simulink model "zynqRadioQPSKRxFPGAAD9361AD9364RetargetSL"  (R2016a)
settings: Solver=FixedStepDiscrete  SolverMode=SingleTasking  StartTime=0.0  StopTime=inf  RelTol=1e-3
PreLoadFcn:
  | sdrzQPSKRxFPGAretarget_params =zynqRadioQPSKRxFPGAAD9361AD9364SL_init;
InitFcn:
  | sdrzQPSKRxFPGAretarget_params = zynqRadioQPSKRxFPGAAD9361AD9364SL_init;
undefined symbols (not defined in the file or in its folder): F
libraries: hdlsllib x3, sdrzblksprivate x1, commsequence2 x1, zc706fmc234_lib x1
CloseFcn:
  | clear sdrzQPSKRxFPGAretarget_params;
Description:
  | This model uses a targeted .bit generated from the sdrzQPSKRxFPGAFMC234 example to receive a QPSK signal using SDR hardware
settings Model: FPTRunName=Active  ModifiedByFormat=The MathWorks Inc.  SimulationMode=accelerator  Creator=The MathWorks, Inc.  LastModifiedBy=The MathWorks Inc.
settings DataIOCC: LimitDataPoints=on  SaveFormat=Structure  SaveOutput=off  SignalLogging=off  DSMLogging=off  SaveTime=off
settings OptimizationCC: BlockReduction=off  ConditionallyExecuteInputs=off  DefaultParameterBehavior=Inlined  ExpressionDepthLimit=2147483647  LocalBlockOutputs=off  SimCompilerOptimization=on
settings DebuggingCC: AlgebraicLoopMsg=error  UnderspecifiedInitializationDetection=Classic  MergeDetectMultiDrivingBlocksExec=none  SolverPrmCheckMsg=warning  MultiTaskDSMMsg=warning  MultiTaskCondExecSysMsg=none  SingleTaskRateTransMsg=error  ParameterPrecisionLossMsg=none  FcnCallInpInsideContextMsg=UseLocalSettings  AllowSymbolicDim=off  StateNameClashWarn=warning
settings HardwareCC: ProdBitPerPointer=32  ProdLargestAtomicFloat=None  ProdIntDivRoundTo=Undefined  ProdEndianess=Unspecified  ProdWordSize=32  ProdHWDeviceType=ASIC/FPGA->ASIC/FPGA  TargetBitPerPointer=64  TargetLongLongMode=on  TargetIntDivRoundTo=Zero  TargetEndianess=LittleEndian  TargetWordSize=64  TargetHWDeviceType=MATLAB Host  ProdEqTarget=off
settings ModelReferenceCC: PropagateSignalLabelsOutOfModel=off
settings RTWCC: CustomSourceCode=|
  | #include <stdio.h>
  | #include <stdlib.h>
settings GRTTargetCC: CombineOutputUpdateFcns=off  GRTInterface=on
settings ConfigComp: CovModelRefEnable=Off  CovSFcnEnable=off

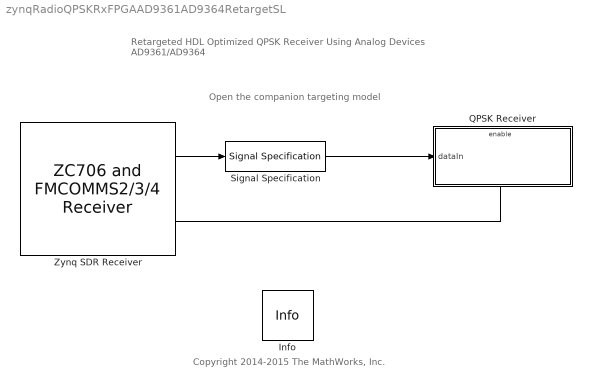
== system zynqRadioQPSKRxFPGAAD9361AD9364RetargetSL ==
  note: Copyright 2014-2015 The MathWorks, Inc.
  note: Retargeted HDL Optimized QPSK Receiver
      | Using Analog Devices AD9361/AD9364
  note: Open the companion targeting model
  Info : sdrzblksprivate/Info  SystemSampleTime=-1
  QPSK Receiver : Subsystem
      mask Display: disp('QPSK Receiver')
  Signal Specification : SignalSpecification  SampleTime=sdrzQPSKRxFPGAretarget_params.Upsampling*sdrzQPSKRxFPGAretarget_params.FrameSize*sdrzQPSKRxFPGAretarget_params.RxBufferedFrames/sdrzQPSKRxFPGAretarget_params.RadioFrontEndSampleRate
  Zynq SDR Receiver : zc706fmc234_lib/ZC706 and  FMCOMMS2//3//4  Receiver  IPAddress=192.168.3.2  CenterFrequencySource=Dialog  CenterFrequency=sdrzQPSKRxFPGAretarget_params.RadioCenterFrequency  GainSource=AGC Slow Attack  Gain=1  ChannelMapping=1  BasebandSampleRate=sdrzQPSKRxFPGAretarget_params.RadioFrontEndSampleRate  EnableBurstMode=on  NumFramesInBurst=20  OutputDataType=int16  SamplesPerFrame=sdrzQPSKRxFPGAretarget_params.Upsampling*sdrzQPSKRxFPGAretarget_params.FrameSize*sdrzQPSKRxFPGAretarget_params.RxBufferedFrames  LostSamplesOutputPort=off  RSSIOutputPort=off  DMATimeoutValue=1  blockMode=Normal  EnableQuadratureTracking=on  EnableRFDCTracking=on  EnableBasebandDCTracking=on  BypassUserLogic=off  ShowAdvancedProperties=on  ShowInternalProperties=off  subDeviceList=zynqReceiver  sdrExecutionMode=HW  dataUDPPort=-1  ctrlUDPPort=-1  SourceSelect=RF data  SourceConfiguration1=1023  FIRCoefficientSize=[ 128; 128 ]  FIRCoefficients=[ 111, -87, 147, -127, -18, -286, -312, -555, -601, -722, -642, -555, -303, -66, 221, 393, 488, 403, 219, -74, -343, -550, -582, -450, -146, 221, 569, 759, 735, 463, 20, -487, -885, -1048, -883, -418, 243, 897, 1340, 1394, 1002, 228, -715, -1549, -1980, -1819, -1028, 217, 1583, 2635, 2980, 2377, 853, -1275, -3435, -4926, -5080, -3454, 40, 5065, 10903, 16581, 21085, 23573, 23573, 21085, 16581, 10903, 5065, 40, -3454, -5080, -4926, -3435, -1275, 853, 2377, 2980, 2635, 1583, 217, -1028, -1819, -1980, -1549, -715, 228, 1002, 1394, 1340, 897, 243, -418, -883, -1048, -885, -487, 20, 463, 735, 759, 569, 221, -146, -450, -582, -550, -343, -74, 219, 403, 488, 393, 221, -66, -303, -555, -642, -722, -601, -555, -312, -286, -18, -127, 147, -87, 111; 382, -200, 711, -41, 645, 36, 346, -194, -119, -543, -472, -646, -404, -312, 45, 197, 413, 346, 241, -93, -373, -680, -755, -689, -356, 51, 515, 795, 870, 609, 136, -488, -1009, -1303, -1191, -712, 69, 885, 1516, 1692, 1336, 468, -662, -1740, -2378, -2329, -1494, -55, 1620, 2995, 3584, 3045, 1368, -1121, -3755, -5708, -6156, -4542, -710, 4969, 11669, 18243, 23486, 26391, 26391, 23486, 18243, 11669, 4969, -710, -4542, -6156, -5708, -3755, -1121, 1368, 3045, 3584, 2995, 1620, -55, -1494, -2329, -2378, -1740, -662, 468, 1336, 1692, 1516, 885, 69, -712, -1191, -1303, -1009, -488, 136, 609, 870, 795, 515, 51, -356, -689, -755, -680, -373, -93, 241, 346, 413, 197, 45, -312, -404, -646, -472, -543, -119, -194, 346, 36, 645, -41, 711, -200, 382 ]  FIRGain=[ 0; -12 ]  FIRDecimInterpFactor=[ 4; 4 ]  AnalogFilterCutoff=[ 2560000; 2560000 ]  FilterPathRates=[ 737280000, 184320000, 61440000, 30720000, 15360000, 3840000; 737280000, 184320000, 61440000, 30720000, 15360000, 3840000 ]  FilterDesignTypeForTx=DefaultFilterFromOther  FilterDesignTypeForRx=DefaultFilter  BISTLoopbackConfig=No Loopback  BISTPRBSMode=PRBS Disable  BISTToneMode=Tone Disable  BISTToneFrequency=F/32  BISTToneLevel=-6  BISTChannelMask=0  DataIsComplex=on  SimulateUsing=Code generation
  wires:
  Zynq SDR Receiver/2 -> QPSK Receiver/Enable
  Zynq SDR Receiver/1 -> Signal Specification/1
  Signal Specification/1 -> QPSK Receiver/1(dataIn)

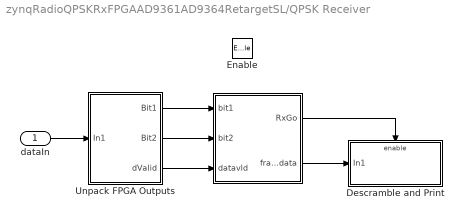
== system zynqRadioQPSKRxFPGAAD9361AD9364RetargetSL/QPSK Receiver ==
  dataIn : Inport  OutDataTypeStr=int16
  Enable : EnablePort
  " " : MATLAB Function  TreatAsAtomicUnit=on
  Descramble and Print : Subsystem  TreatAsAtomicUnit=on
  Unpack FPGA Outputs : Subsystem
  wires:
  Unpack FPGA Outputs/2(Bit2) -> " "/2(bit2)
  Unpack FPGA Outputs/1(Bit1) -> " "/1(bit1)
  Unpack FPGA Outputs/3(dValid) -> " "/3(datavld)
  dataIn/1 -> Unpack FPGA Outputs/1(In1)
  " "/1(RxGo) -> Descramble and Print/Enable
  " "/2(framed_data) -> Descramble and Print/1(In1)

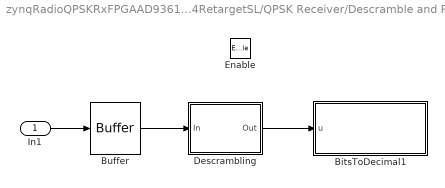
== system zynqRadioQPSKRxFPGAAD9361AD9364RetargetSL/QPSK Receiver/Descramble and Print ==
  In1 : Inport
  Enable : EnablePort
  BitsToDecimal1 : MATLAB Function  TreatAsAtomicUnit=on
  Buffer : Buffer  N=200  TreatMby1Signals=One channel  OutputFrames=off
  Descrambling : Subsystem
      mask Display: disp('Descrambling')
  wires:
  Descrambling/1(Out) -> BitsToDecimal1/1(u)
  In1/1 -> Buffer/1
  Buffer/1 -> Descrambling/1(In)

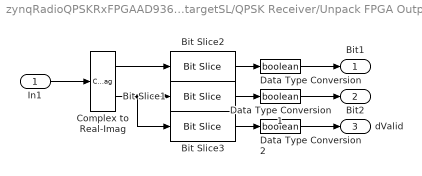
== system zynqRadioQPSKRxFPGAAD9361AD9364RetargetSL/QPSK Receiver/Unpack FPGA Outputs ==
  In1 : Inport
  Bit Slice1 : hdlsllib/HDL Operations/Bit Slice  lidx=0  ridx=0
  Bit Slice2 : hdlsllib/HDL Operations/Bit Slice  lidx=0  ridx=0
  Bit Slice3 : hdlsllib/HDL Operations/Bit Slice  lidx=15  ridx=15
  Complex to Real-Imag : ComplexToRealImag
  Data Type Conversion : DataTypeConversion  OutDataTypeStr=boolean
  Data Type Conversion1 : DataTypeConversion  OutDataTypeStr=boolean
  Data Type Conversion2 : DataTypeConversion  OutDataTypeStr=boolean
  Bit1 : Outport
  Bit2 : Outport  Port=2
  dValid : Outport  Port=3
  wires:
  In1/1 -> Complex to Real-Imag/1
  Complex to Real-Imag/1 -> Bit Slice2/1
  Complex to Real-Imag/2 -> Bit Slice3/1, Bit Slice1/1
  Bit Slice2/1 -> Data Type Conversion/1
  Bit Slice1/1 -> Data Type Conversion1/1
  Bit Slice3/1 -> Data Type Conversion2/1
  Data Type Conversion/1 -> Bit1/1
  Data Type Conversion1/1 -> Bit2/1
  Data Type Conversion2/1 -> dValid/1

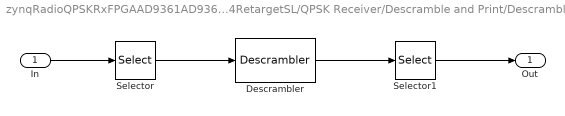
== system zynqRadioQPSKRxFPGAAD9361AD9364RetargetSL/QPSK Receiver/Descramble and Print/Descrambling ==
  In : Inport
  Descrambler : commsequence2/Descrambler  M=2  poly=[1 1 1 0 1]  iniStaSource=Dialog Parameter  ini_sta=[0 0 0 0]  resetViaPort=off
  Selector : Selector  IndexOptions=Index vector (dialog)  Indices=[sdrzQPSKRxFPGAretarget_params.BarkerLength*log2(sdrzQPSKRxFPGAretarget_params.M)+1:sdrzQPSKRxFPGAretarget_params.FrameSize*log2(sdrzQPSKRxFPGAretarget_params.M)]  OutputSizes=1
  Selector1 : Selector  IndexOptions=Index vector (dialog)  Indices=[1:sdrzQPSKRxFPGAretarget_params.MsgLength]  OutputSizes=1
  Out : Outport
  wires:
  Descrambler/1 -> Selector1/1
  Selector1/1 -> Out/1
  In/1 -> Selector/1
  Selector/1 -> Descrambler/1

== matlab function zynqRadioQPSKRxFPGAAD9361AD9364RetargetSL/QPSK Receiver/  ==
  data: RxGo output; framed_data output; bit1 input; bit2 input; datavld input
function [RxGo, framed_data] = dataframer(bit1, bit2, datavld)
%#codegen

persistent  gooddata_from_prev length_prev_good_data


if isempty(gooddata_from_prev)
    gooddata_from_prev = false(8000,1);
    length_prev_good_data = 0;
end

gooddata_current = false(8000,1); % worst case scenario
if any(datavld) % there is some valid data
    % get the valid data from this frame and append it with the previous
    % stored one, if any
    
    %gooddata_current = false(2*sum(datavld),1);
    gooddata_current(1:2:2*sum(datavld)-1) = bit1(logical(datavld));
    gooddata_current(2:2:2*sum(datavld))   = bit2(logical(datavld));
    % append with prev good data
    data_tmp = [gooddata_from_prev(1:length_prev_good_data);gooddata_current(1:2*sum(datavld))];
    if length(data_tmp) > 8000
        framed_data = data_tmp(1:8000);
        RxGo = 1;
        gooddata_length_athand = length(data_tmp);
        datalen_fornext = gooddata_length_athand -8000;
        gooddata_from_prev(1:datalen_fornext) = data_tmp(8001:8001+datalen_fornext-1);
        length_prev_good_data = datalen_fornext;
    elseif length(data_tmp) == 8000
        framed_data = data_tmp(1:8000);
        RxGo = 1;
        gooddata_from_prev =  false(8000,1);
        length_prev_good_data = 0;
    else % less than 8000
        gooddata_length_athand = length(data_tmp);
        datalen_fornext = gooddata_length_athand;      
        gooddata_from_prev(1:gooddata_length_athand) = data_tmp(1:gooddata_length_athand);
        length_prev_good_data = datalen_fornext;
        framed_data = false(8000,1); % garbage
        RxGo = 0;
    end
    
else % none of the data is valid
    RxGo = 0;
    framed_data = false(8000,1); %just send the data through
    gooddata_from_prev = false(8000,1);
    length_prev_good_data = 0;
end

== matlab function zynqRadioQPSKRxFPGAAD9361AD9364RetargetSL/QPSK Receiver/Descramble and Print/BitsToDecimal1 ==
  data: u input
function BitsToASCII(u)
% Convert bits to ASCII message.

persistent package_counter;
persistent error_counter;
if isempty(package_counter)
    package_counter = 0;
    error_counter   = 0;
end

coder.extrinsic('disp')
coder.extrinsic('num2str')

aa = de2bi(int8('Hello world 0'),7,'left-msb');
bits_ref = double(reshape(aa.',1,[]));
bits_ref = bits_ref(:);

error_counter   = error_counter   + sum(abs(bits_ref - u(1:91)));
package_counter = package_counter + 1;

% Convert binary-valued column vector to 7-bit decimal values.
w = [64 32 16 8 4 2 1]; % binary digit weighting
Nbits = numel(u);
Ny = Nbits/7;
y = zeros(1,Ny);
for i = 0:Ny-1
    y(i+1) = w*u(7*i+(1:7));
end

% Display ASCII message to command window
disp(char(y));
